simulink model "Mmc"  (R2024b)
settings: Solver=ode23t  StartTime=0.0  StopTime=3  FixedStep=Ts_Power
values from neighbouring files (symbols this model uses):
  alpha_i = (pi/2 - 75/180*pi) / tau_sw    (= 26179.9387799)    [MmcParameters.m]
  C_PM = 6e-3    (= 0.006)    [MmcParameters.m]
  eta = N*delta_wmax*V0^2/(P_rated*sin(phi_r)-Q_rated*cos(phi_r))    [MmcParameters.m]
  Fnom = 50    [MmcParameters.m]
  fs = 400    [MmcParameters.m]
  I_b = Snom/Vnom_AC/sqrt(3)    [MmcParameters.m]
  Ipp_b = Snom/Vnom_AC/sqrt(3/2)    [MmcParameters.m]
  kicir = R0*alpha_ic    (= 2617.99387799)    [MmcParameters.m]
  kiout = R*alpha_i    (= 1308.996939)    [MmcParameters.m]
  kip = 500    [MmcParameters.m]
  kpcir = L0*alpha_ic    (= 416.666666667)    [MmcParameters.m]
  kpout = L*alpha_i    (= 208.333333333)    [MmcParameters.m]
  kpp = 1.5    [MmcParameters.m]
  L = L0/2    (= 0.00795774715459)    [MmcParameters.m]
  L0 = .25 * L_b    (= 0.0159154943092)    [MmcParameters.m]
  mu = eta/2/N/V0^2/(Vmax^2-V0^2)*(P_rated*cos(phi_r)+Q_rated*sin(phi_r))    [MmcParameters.m]
  Nb_PM = 20    [MmcParameters.m]
  phi_r = pi/2    (= 1.57079632679)    [MmcParameters.m]
  R0 = .1    (= 0.1)    [MmcParameters.m]
  SCR = 1.2    [MmcParameters.m]
  SigmaM = 10    [MmcParameters.m]
  Snom = 80e6    (= 80000000)    [MmcParameters.m]
  Ts_Power = 1e-5    (= 1e-05)    [MmcParameters.m]
  V0 = 1    [MmcParameters.m]
  V_b = Vnom_AC    (= 40000)    [MmcParameters.m]
  VDCm = 48e3    (= 48000)    [MmcParameters.m]
  VDCp = 48e3    (= 48000)    [MmcParameters.m]
  Vnom_AC = 40e3    (= 40000)    [MmcParameters.m]
  Vnom_PM = 4.8e3    (= 4800)    [MmcParameters.m]
  w_b = 2*pi*Fnom    (= 314.159265359)    [MmcParameters.m]
undefined symbols (not defined in the file or in its folder): DiscIntNeverNeededParam, Lac, Rac
libraries: spsCurrentMeasurementLib x7, spsHalfBridgeMMCLib x6, spsSeriesRLCBranchLib x6, slpidlib x6, eePwmGeneratorMultilevel x6, spsabctodq0Lib x3, spsMeanLib x2, spsDCVoltageSourceLib x2, spsThreePhaseVIMeasurementLib x2, spsPLL3phLib x2, spsdq0toabcLib x2, spsabctoAlphaBetaZeroLib x2
(part 1 of 2)
settings Model: Creator=The MathWorks, Inc.  LastModifiedBy=smile
settings SolverCC: AlgebraicLoopSolver=TrustRegion
settings DataIOCC: SaveFormat=StructureWithTime  SaveOutput=off  SignalLogging=off  DSMLogging=off  SaveTime=off  ReturnWorkspaceOutputs=off
settings OptimizationCC: ExpressionDepthLimit=2147483647  LifeSpan=inf
settings DebuggingCC: UnderspecifiedInitializationDetection=Classic  MergeDetectMultiDrivingBlocksExec=none  SolverPrmCheckMsg=warning  FcnCallInpInsideContextMsg=warning  UnconnectedInputMsg=warning  UnconnectedOutputMsg=warning  UnconnectedLineMsg=warning  AllowSymbolicDim=off  StateNameClashWarn=warning  SFUnexpectedBacktrackingDiag=warning  SFNoUnconditionalDefaultTransitionDiag=warning  SFExecutionAtInitializationDiag=none  ArithmeticOperatorsInVariantConditions=warning
settings HardwareCC: ProdBitPerPointer=32  ProdBitPerSizeT=32  ProdBitPerPtrDiffT=32  ProdLargestAtomicFloat=None  ProdIntDivRoundTo=Undefined  ProdEndianess=Unspecified  ProdWordSize=32  ProdHWDeviceType=32-bit Generic
settings ModelReferenceCC: EnableRefExpFcnMdlSchedulingChecks=on  PropagateSignalLabelsOutOfModel=off
settings SFSimCC: SimUseLocalCustomCode=off  CustomCodeUndefinedFunction=UseInterfaceOnly
settings RTWCC: RTWUseLocalCustomCode=off  GPUComputeCapability=3.5
settings CodeAppCC: StateflowObjectComments=on
settings GRTTargetCC: TargetLangStandard=C89/C90 (ANSI)  CombineOutputUpdateFcns=off  GRTInterface=on
settings ConfigComp: CovMetricSettings=dw  CovSaveCumulativeToWorkspaceVar=on  CovSaveSingleToWorkspaceVar=on  CovExternalEMLEnable=off
settings SimscapeCC: SimscapeNormalizeSystem=off  SimscapeNominalValues={1, 'bar'; 1, 'cm^3/s'; 1, 'bar*kg/s'; 1, 'kJ/kg'; 1, 'kW'; }

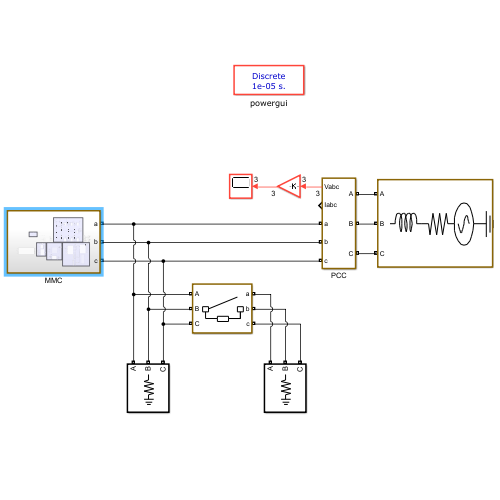
[thumbnail: Simulink's stored preview of the top-level diagram]
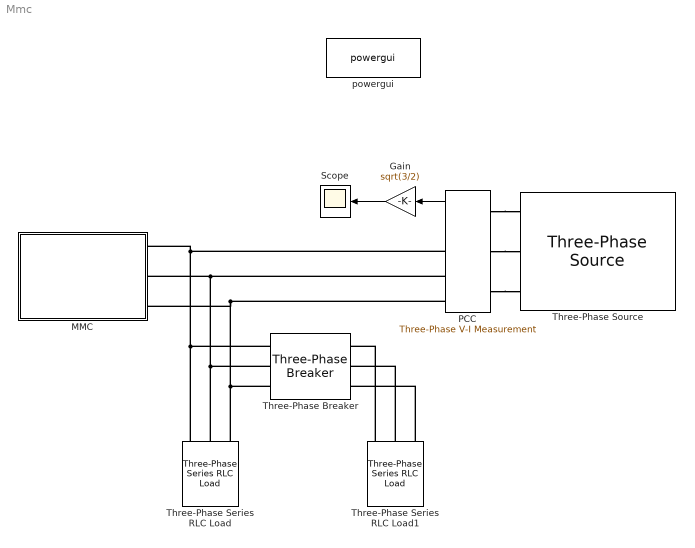
== system Mmc ==
  Gain : Gain  Gain=sqrt(3/2)
  MMC : Subsystem
  PCC : spsThreePhaseVIMeasurementLib/Three-Phase V-I Measurement  VoltageMeasurement=phase-to-ground  SetLabelV=off  LabelV=Vabc  Vpu=off  VpuLL=off  CurrentMeasurement=yes  SetLabelI=off  LabelI=Iabc  Ipu=off  Pbase=Snom  Vbase=Vnom_AC  OutputType=Complex  PhasorSimulation=off  PSBequivalent=0
  Scope : Scope
  Three-Phase Series RLC Load : spsThreePhaseSeriesRLCLoadLib/Three-Phase Series RLC Load  LConnTagsString=A|B|C  Configuration=Y (grounded)  NominalVoltage=Vnom_AC  Vabc=[1e3 1e3 1e3]  Vabcp=[1e3 1e3 1e3]  NominalFrequency=Fnom  UnbalancedPower=off  ActivePower=1e-6  InductivePower=0  CapacitivePower=0  Pabc=[10e3 9e3 11e3]  QLabc=[100 90 110]  QCabc=[100 90 110]  Pabcp=[10e3 9e3 11e3]  QLabcp=[100 90 110]  QCabcp=[100 90 110]  Measurements=None  LoadType=constant Z
  Three-Phase Series RLC Load1 : spsThreePhaseSeriesRLCLoadLib/Three-Phase Series RLC Load  LConnTagsString=A|B|C  Configuration=Y (grounded)  NominalVoltage=Vnom_AC  Vabc=[1e3 1e3 1e3]  Vabcp=[1e3 1e3 1e3]  NominalFrequency=Fnom  UnbalancedPower=off  ActivePower=Snom/1  InductivePower=0  CapacitivePower=0  Pabc=[10e3 9e3 11e3]  QLabc=[100 90 110]  QCabc=[100 90 110]  Pabcp=[10e3 9e3 11e3]  QLabcp=[100 90 110]  QCabcp=[100 90 110]  Measurements=None  LoadType=constant PQ
  Three-Phase Breaker : spsThreePhaseBreakerLib/Three-Phase Breaker  InitialState=open  SwitchA=on  SwitchB=on  SwitchC=on  SwitchTimes=[2]  External=off  BreakerResistance=1e-9  SnubberResistance=1e9  SnubberCapacitance=inf  Measurements=None
  Three-Phase Source : spsThreePhaseSourceLib/Three-Phase Source  InternalConnection=Yg  VoltagePhases=off  Voltage=Vnom_AC/1  PhaseAngle=0  Voltage_phases=[25e3 25e3 25e3]/sqrt(3)  PhaseAngles_phases=[0 -120 +120]  Frequency=Fnom  NonIdealSource=on  SpecifyImpedance=on  Resistance=Rac/1e9  Inductance=Lac/1e4  ShortCircuitLevel=SCR*Snom  BaseVoltage=Vnom_AC  XRratio=7  BusType=swing  Pref=10e3  Qref=0  Prefabc=[10e3, 10e3, 10e3]  Qrefabc=[0, 0, 0]  Qmin=-inf  Qmax=inf
  powergui : sps_lib/powergui  Priority=1  SimulationMode=Discrete  SampleTime=Ts_Power  frequency=60  Iterations=50  frequencyindice=50  Pbase=100e6  ErrMax=1e-4  UnitsV=kV  UnitsW=MW  buscounter=0  FunctionMessages=off  echomessages=off  EnableUseOfTLC=off  CurrentSourceSwitches=off  DisableSnubberDevices=off  DisableRonSwitches=off  DisableVfSwitches=off  DisplayEquations=off  AutomaticDiscreteSolvers=off  SolverType=Tustin/Backward Euler (TBE)  Interpol=off  ExternalGateDelay=off  methode=off  Ts=10  x0status=blocks  SPID=off  SwTol=0  HookPort=off  NonlinearTolerance=1e-4  nMaxIteration=100  ContinueOnMaxIteration=off  RestoreLinks=warning  ResistiveCurrentMeasurement=off  Frange=[0:2:500]  Ylog=off  Xlog=on  ShowGrid=off  save=off  variable=ZData  structure=Vout  ZoomFFT=on  StartTime=0.15  cycles=2  DisplayStyle=1  fundamental=50  FreqAxis=on  MaxFrequency=6000  frequencyindicesteady=1  RmsSteady=1  display=off
  wires:
  PCC/1 -> Gain/1
  Gain/1 -> Scope/1
  connections:
  Three-Phase Series RLC Load/LConn1 -- Three-Phase Breaker/LConn1 -- PCC/RConn1 -- MMC/LConn1
  Three-Phase Series RLC Load/LConn2 -- Three-Phase Breaker/LConn2 -- PCC/RConn2 -- MMC/LConn2
  Three-Phase Series RLC Load/LConn3 -- Three-Phase Breaker/LConn3 -- PCC/RConn3 -- MMC/LConn3
  Three-Phase Series RLC Load1/LConn1 -- Three-Phase Breaker/RConn1
  Three-Phase Series RLC Load1/LConn2 -- Three-Phase Breaker/RConn2
  Three-Phase Series RLC Load1/LConn3 -- Three-Phase Breaker/RConn3
  PCC/LConn1 -- Three-Phase Source/RConn1
  PCC/LConn2 -- Three-Phase Source/RConn2
  PCC/LConn3 -- Three-Phase Source/RConn3

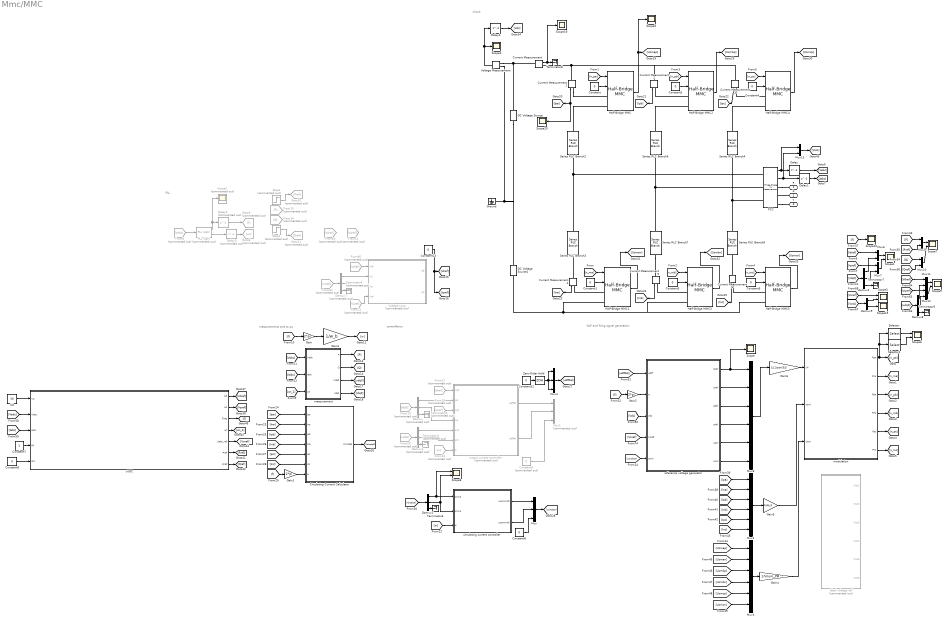
== system Mmc/MMC ==
  note: controllerws
  note: circuit
  note: NLP and firing signal generation
  note: measurements and to pu
  note: PLL
  Circulating Current Calculator : Subsystem
  Constant{,1..6,8,12..13} (10 alike) : Constant  Value=0
  Constant7 : Constant
  Constant9 : Constant  Commented=on  Value=0
  Current Measurement{,1..6} (7 alike) : spsCurrentMeasurementLib/Current Measurement  PhasorSimulation=off  OutputType=Complex  PSBequivalent=0
  DC Voltage Source : spsDCVoltageSourceLib/DC Voltage Source  Amplitude=VDCp  Measurements=None
  DC Voltage Source1 : spsDCVoltageSourceLib/DC Voltage Source  Amplitude=VDCm  Measurements=None
  Delay : Delay  DelayLength=1  SampleTime=Ts_Power
  Delay1 : Delay  DelayLength=1  SampleTime=Ts_Power
  Delay2 : Delay  Commented=on  DelayLength=1  SampleTime=Ts_Power
  Delay3 : Delay  Commented=on  DelayLength=1  SampleTime=Ts_Power
  Delay4 : Delay  DelayLength=1  InputProcessing=Columns as channels (frame based)
  Demux : Demux  Commented=on  Outputs=3
  Demux1 : Demux  Commented=on  Outputs=3
  Demux2 : Demux  Outputs=3
  Demux3 : Demux  Outputs=3
  Demux7 : Demux  Commented=on  Outputs=3
  Demux8 : Demux  Outputs=3
  Demux9 : Demux  Outputs=2
  From13 : From  Commented=on  GotoTag=w
  From15 : From  Commented=on  GotoTag=P
  From16 : From  Commented=on  GotoTag=Q
  From17 : From  Commented=on  GotoTag=idref
  From18 : From  Commented=on  GotoTag=iqref
  From19 : From  Commented=on  GotoTag=idq0
  From20 : From  Commented=on  GotoTag=udq0
  From60 : From  Commented=on  GotoTag=Vdref
  From61 : From  Commented=on  GotoTag=Vqref
  From62 : From  Commented=on  GotoTag=udq0
  From66 : From  Commented=on  GotoTag=Vdref
  From72 : From  Commented=on  GotoTag=Vqref
  From8 : From  Commented=on  GotoTag=Vabc
  Gain : Gain  Gain=2*pi
  Gain1 : Gain  Gain=2*pi
  Gain2 : Gain  Gain=2*pi
  Gain3 : Gain  Gain=1/w_b
  Gain4 : Gain  Gain=1/Vnom_PM
  Gain5 : Gain  Gain=1/Ipp_b
  Gain6 : Gain  Gain=1/1.2/sqrt(3/2)
  Goto10 : Goto  Commented=on  GotoTag=Pref
  Goto11 : Goto  Commented=on  GotoTag=Qref
  Goto8 : Goto  Commented=on  GotoTag=wt
  Goto9 : Goto  Commented=on  GotoTag=f
  Ground : spsGroundLib/Ground  LConnTagsString=a
  Half-Bridge MMC{,1..5} (6 alike) : spsHalfBridgeMMCLib/Half-Bridge MMC  ModelType=Switching devices  n=Nb_PM  C=C_PM  Vc_Initial=Vc_Initial  Ron=Ron  Rs=Rs  Cs=Cs  Ron_Diode=1e-3  Rs_Diode=1e6  Cs_Diode=inf  Vf_Diode=1e-3  Rs_CurrentSource=inf  Ts=10e-6
      settings: LibrarySourceBlock=sps_lib/Power Electronics/Half-Bridge MMC
  Ideal voltage ref : Subsystem  Commented=on
  Mux : Mux  Inputs=3
  Mux1 : Mux  Commented=on  Inputs=3
  Mux{6..7,9..13} (7 alike) : Mux  Inputs=2
  Mux2 : Mux  Inputs=6
  Mux3 : Mux  Inputs=6
  Mux4 : Mux  Inputs=3
  Mux8 : Mux  Inputs=6
  PCC : spsThreePhaseVIMeasurementLib/Three-Phase V-I Measurement  VoltageMeasurement=phase-to-ground  SetLabelV=off  LabelV=Vabc  Vpu=on  VpuLL=off  CurrentMeasurement=yes  SetLabelI=off  LabelI=Iabc  Ipu=on  Pbase=Snom  Vbase=Vnom_AC  OutputType=Complex  PhasorSimulation=off  PSBequivalent=0
  PLL (3ph) : spsPLL3phLib/PLL (3ph)  Commented=on  Fmin=45  Par_Init=[0, 50]  ParK=[9.2/.2 (4.6/.2/.7)^2 0]  TcD=1e-4  MaxRateChangeFreq=12  FilterCutOffFreq=50  Ts=0  AGC=on
  Scope{,4..5,10,15,19..20} (7 alike) : Scope
  Scope{1,3,6..9} (6 alike) : Scope  NumInputPorts=2
  Scope2 : Scope  Commented=on
  Selector : Selector  InputPortWidth=2*Nb_PM  IndexOptions=Index vector (dialog)  Indices=[1]  OutputSizes=1
  Selector1 : Selector  InputPortWidth=2*Nb_PM  IndexOptions=Index vector (dialog)  Indices=[Nb_PM]  OutputSizes=1
  Series RLC Branch{2..4,6..8} (6 alike) : spsSeriesRLCBranchLib/Series RLC Branch  LConnTagsString=__new0  RConnTagsString=__new0  BranchType=RL  Resistance=R0  Inductance=L0  SetiL0=off  InitialCurrent=0  Capacitance=1e-6  Setx0=off  InitialVoltage=0  Measurements=None
  Step2 : Step  Commented=on  Time=.3  Before=-.1  After=.7  SampleTime=Ts_Power
  Step3 : Step  Commented=on  Time=.7  Before=-.1  After=0.7  SampleTime=Ts_Power
  Terminator2 : Terminator  Commented=on
  Terminator3 : Terminator  Commented=on
  Terminator4 : Terminator  Commented=on
  Terminator{6..9} (4 alike) : Terminator
  U0 : Constant  Value=V0  SampleTime=Ts_Power
  Voltage Loop : Subsystem  Commented=on
  Voltage Measurement : spsVoltageMeasurementLib/Voltage Measurement  PhasorSimulation=off  OutputType=Complex  PSBequivalent=0
  Zero-Order Hold : ZeroOrderHold  SampleTime=Ts_Power
  circulating current controller : Subsystem
  measurement : Subsystem
  modulation : Subsystem
  output current controller : Subsystem  Commented=on
  reference voltage generator : Subsystem
  uVOC : Subsystem
  a : PMIOPort  Side=Left
  b : PMIOPort  Port=2  Side=Left
  c : PMIOPort  Port=3  Side=Left
  wires:
  Constant4/1 -> Half-Bridge MMC4/2
  [n_pc] -> Half-Bridge MMC4/1
  [n_pb] -> Half-Bridge MMC2/1
  [n_pa] -> Half-Bridge MMC/1
  [n_mb] -> Half-Bridge MMC3/1
  Constant1/1 -> Half-Bridge MMC1/2
  Constant3/1 -> Half-Bridge MMC3/2
  Half-Bridge MMC/1 -> Scope5/1, [Usmap]
  Constant2/1 -> Half-Bridge MMC2/2
  Constant/1 -> Half-Bridge MMC/2
  [n_ma] -> Half-Bridge MMC1/1
  Constant5/1 -> Half-Bridge MMC5/2
  [n_mc] -> Half-Bridge MMC5/1
  PCC/1 -> Mux13/1, Delay/1
  PCC/2 -> Mux13/2, Delay1/1
  [Vabc] -> measurement/1(Vabc)
  [Iabc] -> measurement/2(Iabc)
  From8/1 -> PLL (3ph)/1
  PLL (3ph)/2 -> Delay3/1
  [wt_2] -> measurement/3(wt)
  PLL (3ph)/1 -> Scope2/1, Delay2/1
  [f] -> Gain/1
  Gain/1 -> Gain3/1
  Gain3/1 -> [w]
  From13/1 -> output current controller/7(w)
  circulating current controller/1(ucommd*) -> Mux/1
  circulating current controller/2(ucommq*) -> Mux/2
  Constant6/1 -> Mux/3
  measurement/1(P) -> [P]
  From17/1 -> output current controller/1(ivd*)
  From18/1 -> output current controller/3(ivq*)
  measurement/3(Vdq0) -> [udq0]
  measurement/4(Idq0) -> [idq0]
  From19/1 -> Demux/1
  Demux/2 -> output current controller/4(ivq)
  Demux/1 -> output current controller/2(ivd)
  Demux/3 -> Terminator2/1
  From20/1 -> Demux1/1
  Demux1/1 -> output current controller/5(uvd)
  Demux1/2 -> output current controller/6(uvq)
  Demux1/3 -> Terminator3/1
  [w] -> circulating current controller/3(w)
  Current Measurement1/1 -> Scope20/1, [Ipa]
  Current Measurement2/1 -> [Ipb]
  Current Measurement3/1 -> [Ipc]
  Current Measurement4/1 -> [Ina]
  Current Measurement5/1 -> [Inb]
  Current Measurement6/1 -> [Inc]
  [Ipa] -> Circulating Current Calculator/1(ipa)
  [Ina] -> Circulating Current Calculator/2(ina)
  [Ipb] -> Circulating Current Calculator/3(ipb)
  [Inb] -> Circulating Current Calculator/4(inb)
  [Ipc] -> Circulating Current Calculator/5(ipc)
  [Inc] -> Circulating Current Calculator/6(inc)
  [f] -> Gain1/1
  Gain1/1 -> Circulating Current Calculator/7(w)
  Circulating Current Calculator/1(icircdq0) -> [Icircdq0]
  [Icircdq0] -> Demux2/1
  Demux2/1 -> Scope8/1, circulating current controller/1(Icircd)
  Demux2/2 -> circulating current controller/2(Icircq), Scope8/2
  Demux2/3 -> Terminator6/1
  Constant9/1 -> Mux1/3
  Gain2/1 -> reference voltage generator/2(w)
  [f] -> Gain2/1
  measurement/2(Q) -> [Q]
  Step3/1 -> Goto11/1
  Delay/1 -> [Vabc]
  Delay1/1 -> [Iabc]
  Delay2/1 -> Goto9/1
  Delay3/1 -> Goto8/1
  modulation/1(Ppa) -> [n_pa], Selector1/1, Selector/1
  modulation/2(Pna) -> [n_ma]
  modulation/3(Ppb) -> [n_pb]
  modulation/4(Pnb) -> [n_mb]
  modulation/5(Ppc) -> [n_pc]
  modulation/6(Pnc) -> [n_mc]
  Step2/1 -> Goto10/1
  [idq0] -> Demux3/1
  Demux3/3 -> Terminator7/1
  [idref] -> Mux6/1
  Demux3/1 -> Mux6/2
  [iqref] -> Mux7/1
  Demux3/2 -> Mux7/2
  Mux/1 -> [ucircdq0]
  [P] -> Mux9/1
  [Pref] -> Mux9/2
  [Q] -> Mux10/1
  [Qref] -> Mux10/2
  reference voltage generator/1(upa*) -> Scope/1, Mux8/1
  reference voltage generator/2(una*) -> Mux8/2
  reference voltage generator/3(upb*) -> Mux8/3
  reference voltage generator/4(unb*) -> Mux8/4
  reference voltage generator/5(upc*) -> Mux8/5
  reference voltage generator/6(unc*) -> Mux8/6
  [Ipa] -> Mux2/1
  [Ina] -> Mux2/2
  [Ipb] -> Mux2/3
  [Inb] -> Mux2/4
  [Ipc] -> Mux2/5
  [Inc] -> Mux2/6
  Mux2/1 -> Gain5/1
  Current Measurement/1 -> Scope19/1, Terminator8/1
  Half-Bridge MMC2/1 -> [Usmbp]
  Half-Bridge MMC4/1 -> [Usmcp]
  Half-Bridge MMC1/1 -> [Usman]
  Half-Bridge MMC3/1 -> [Usmbn]
  Half-Bridge MMC5/1 -> [Usmcn]
  [Usmap] -> Mux3/1
  [Usman] -> Mux3/2
  [Usmbp] -> Mux3/3
  [Usmbn] -> Mux3/4
  [Usmcp] -> Mux3/5
  Mux3/1 -> Gain4/1
  [Usmcn] -> Mux3/6
  Gain4/1 -> modulation/3(Usm)
  Gain5/1 -> modulation/2(Iarm)
  Selector/1 -> Scope6/1
  Selector1/1 -> Scope6/2
  Voltage Measurement/1 -> Delay4/1, Scope4/1
  Delay4/1 -> [Vdc]
  Demux7/1 -> Voltage Loop/2(Vd)
  From62/1 -> Demux7/1
  Demux7/3 -> Terminator4/1
  Demux7/2 -> Voltage Loop/3(Vq)
  From66/1 -> Voltage Loop/1(Vd*)
  Mux6/1 -> Scope1/1
  Mux7/1 -> Scope1/2
  Mux9/1 -> Scope7/1
  Mux10/1 -> Scope7/2
  [udq0] -> Demux8/1
  Demux8/3 -> Terminator9/1
  [Vdref] -> Mux11/1
  Demux8/1 -> Mux11/2
  [Vqref] -> Mux12/1
  Demux8/2 -> Mux12/2
  Mux11/1 -> Scope9/1
  Mux12/1 -> Scope9/2
  Mux13/1 -> [VoIo]
  [VoIo] -> Demux9/1
  [Voref] -> Scope3/1
  Demux9/1 -> Scope3/2
  [f] -> Scope10/1
  From72/1 -> Voltage Loop/4(Vq*)
  [Voref] -> reference voltage generator/4(Voref)
  [ucircdq0] -> reference voltage generator/5(ucirc)
  [udiffdq0] -> reference voltage generator/1(udiff)
  [Vdc] -> reference voltage generator/3(Vdc)
  Demux9/2 -> Scope15/1
  output current controller/1(udiffd*) -> Mux1/1
  output current controller/2(udiffq*) -> Mux1/2
  Mux4/1 -> [udiffdq0]
  Constant13/1 -> [idref], [iqref]
  Mux8/1 -> Gain6/1
  U0/1 -> uVOC/1(V0)
  [Vabc] -> uVOC/2(Vabc)
  [Iabc] -> uVOC/3(Iabc)
  Constant7/1 -> uVOC/4(P0)
  Constant8/1 -> uVOC/5(Q0)
  uVOC/1(Ud) -> [Vdref]
  uVOC/6(Pref) -> [Pref]
  uVOC/2(Uq) -> [Vqref]
  uVOC/3(Freq) -> [f]
  uVOC/4(wt) -> [wt_2]
  uVOC/7(Qref) -> [Qref]
  uVOC/5(Uabc_ref) -> [Voref]
  Gain6/1 -> modulation/1(U*)
  Constant12/1 -> Zero-Order Hold/1
  Zero-Order Hold/1 -> Mux4/3, Mux4/1, Mux4/2
  connections:
  Half-Bridge MMC5/LConn2 -- Half-Bridge MMC3/LConn2 -- Half-Bridge MMC1/LConn2 -- DC Voltage Source1/LConn1
  Series RLC Branch4/LConn1 -- Half-Bridge MMC4/LConn2
  Current Measurement/RConn1 -- Current Measurement2/LConn1 -- Current Measurement3/LConn1 -- Current Measurement1/LConn1
  Series RLC Branch8/LConn1 -- PCC/LConn3 -- Series RLC Branch4/RConn1
  Series RLC Branch2/LConn1 -- Half-Bridge MMC/LConn2
  Series RLC Branch3/LConn1 -- Series RLC Branch2/RConn1 -- PCC/LConn1
  Series RLC Branch6/LConn1 -- Half-Bridge MMC2/LConn2
  Series RLC Branch7/LConn1 -- Series RLC Branch6/RConn1 -- PCC/LConn2
  PCC/RConn1 -- a/RConn1
  b/RConn1 -- PCC/RConn2
  PCC/RConn3 -- c/RConn1
  Current Measurement/LConn1 -- DC Voltage Source/RConn1 -- Voltage Measurement/LConn1
  Current Measurement1/RConn1 -- Half-Bridge MMC/LConn1
  Half-Bridge MMC2/LConn1 -- Current Measurement2/RConn1
  Half-Bridge MMC4/LConn1 -- Current Measurement3/RConn1
  Half-Bridge MMC1/LConn1 -- Current Measurement4/RConn1
  Current Measurement4/LConn1 -- Series RLC Branch3/RConn1
  Series RLC Branch7/RConn1 -- Current Measurement5/LConn1
  Half-Bridge MMC3/LConn1 -- Current Measurement5/RConn1
  Current Measurement6/LConn1 -- Series RLC Branch8/RConn1
  Half-Bridge MMC5/LConn1 -- Current Measurement6/RConn1
  DC Voltage Source1/RConn1 -- DC Voltage Source/LConn1 -- Voltage Measurement/LConn2 -- Ground/LConn1

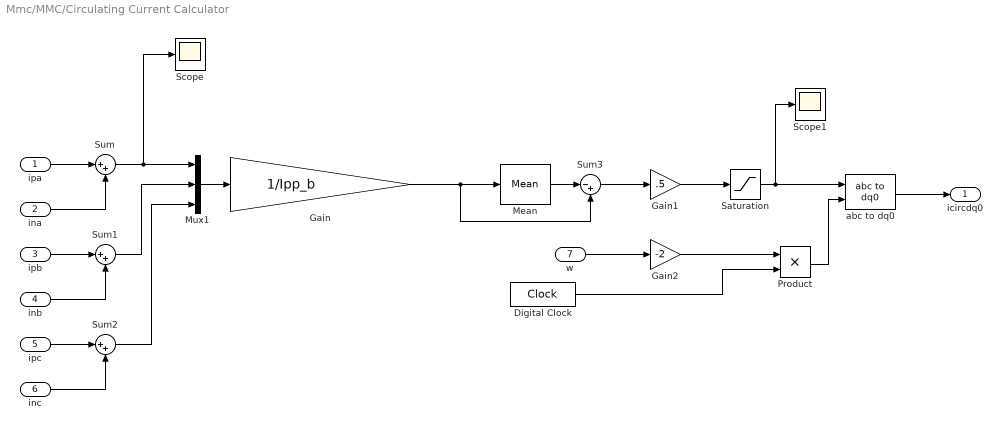
== system Mmc/MMC/Circulating Current Calculator ==
  ipa : Inport
  ina : Inport  Port=2
  ipb : Inport  Port=3
  inb : Inport  Port=4
  ipc : Inport  Port=5
  inc : Inport  Port=6
  w : Inport  Port=7
  Digital Clock : DigitalClock  SampleTime=Ts_Power
  Gain : Gain  Gain=1/Ipp_b
  Gain1 : Gain  Gain=.5
  Gain2 : Gain  Gain=-2
  Mean : spsMeanLib/Mean  Freq=Fnom*2*2  Vinit=0  Ts=Ts_Power
  Mux1 : Mux  Inputs=3
  Product : Product
  Saturation : Saturate  UpperLimit=1.2  LowerLimit=-1.2
  Scope : Scope
  Scope1 : Scope
  Sum : Sum  Inputs=|++
  Sum1 : Sum  Inputs=|++
  Sum2 : Sum  Inputs=|++
  Sum3 : Sum  Inputs=|-+
  abc to dq0 : spsabctodq0Lib/abc to dq0  Alignment=90 degrees behind phase A axis
  icircdq0 : Outport
  wires:
  Sum2/1 -> Mux1/3
  ina/1 -> Sum/2
  Mux1/1 -> Gain/1
  ipb/1 -> Sum1/1
  Sum/1 -> Scope/1, Mux1/1
  Sum1/1 -> Mux1/2
  ipc/1 -> Sum2/1
  inb/1 -> Sum1/2
  ipa/1 -> Sum/1
  inc/1 -> Sum2/2
  Gain1/1 -> Saturation/1
  abc to dq0/1 -> icircdq0/1
  w/1 -> Gain2/1
  Gain2/1 -> Product/1
  Digital Clock/1 -> Product/2
  Product/1 -> abc to dq0/2
  Mean/1 -> Sum3/1
  Sum3/1 -> Gain1/1
  Gain/1 -> Mean/1, Sum3/2
  Saturation/1 -> Scope1/1, abc to dq0/1

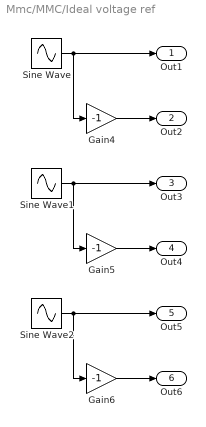
== system Mmc/MMC/Ideal voltage ref ==
  Gain4 : Gain  Gain=-1
  Gain5 : Gain  Gain=-1
  Gain6 : Gain  Gain=-1
  Sine Wave : Sin  Amplitude=sqrt(3/2)  Frequency=50*2*pi  SampleTime=Ts_Power
  Sine Wave1 : Sin  Amplitude=Vnom_AC*sqrt(2/3)/Vnom_PM/Nb_PM  Frequency=50*2*pi  Phase=4*pi/3  SampleTime=Ts_Power
  Sine Wave2 : Sin  Amplitude=Vnom_AC*sqrt(2/3)/Vnom_PM/Nb_PM  Frequency=50*2*pi  Phase=2*pi/3  SampleTime=Ts_Power
  Out1 : Outport
  Out2 : Outport  Port=2
  Out3 : Outport  Port=3
  Out4 : Outport  Port=4
  Out5 : Outport  Port=5
  Out6 : Outport  Port=6
  wires:
  Gain4/1 -> Out2/1
  Sine Wave1/1 -> Out3/1, Gain5/1
  Sine Wave2/1 -> Out5/1, Gain6/1
  Sine Wave/1 -> Out1/1, Gain4/1
  Gain6/1 -> Out6/1
  Gain5/1 -> Out4/1

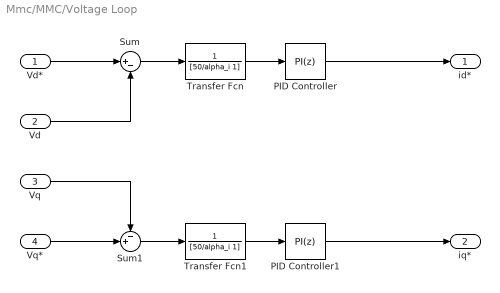
== system Mmc/MMC/Voltage Loop ==
  Vd* : Inport
  Vd : Inport  Port=2
  Vq : Inport  Port=3
  Vq* : Inport  Port=4
  PID Controller : slpidlib/PID Controller  Controller=PI  Form=Parallel  TimeDomain=Discrete-time  UseExternalTs=off  SampleTime=-1  IntegratorMethod=Forward Euler  FilterMethod=Forward Euler  ControllerParametersSource=internal  P=kpp  I=kip  UseKiTs=off  D=0  UseExternalDerivativeSource=off  N=100  UseFilter=on  TunerSelectOption=Transfer Function Based (PID Tuner App)  InitialConditionSource=internal  InitialConditionForIntegrator=0  InitialConditionForFilter=0  DifferentiatorICPrevScaledInput=0  ExternalReset=none  TrackingMode=off  Kt=1  LimitOutput=off  SatLimitsSource=internal  UpperSaturationLimit=inf  LowerSaturationLimit=-inf  LinearizeAsGain=on  AntiWindupMode=none  Kb=1  LimitIntegrator=off  UpperIntegratorSaturationLimit=inf  LowerIntegratorSaturationLimit=-inf  POutMin=[]  POutMax=[]  IOutMin=[]  IOutMax=[]  DOutMin=[]  DOutMax=[]  NOutMin=[]  NOutMax=[]  SumOutMin=[]  SumOutMax=[]  SaturationOutMin=[]  SaturationOutMax=[]  PParamMin=[]  PParamMax=[]  IParamMin=[]  IParamMax=[]  DParamMin=[]  DParamMax=[]  NParamMin=[]  NParamMax=[]  KbParamMin=[]  KbParamMax=[]  KtParamMin=[]  KtParamMax=[]  KbOutMin=[]  KbOutMax=[]  KtOutMin=[]  KtOutMax=[]  IntegratorOutMin=[]  IntegratorOutMax=[]  FilterOutMin=[]  FilterOutMax=[]  SumI1OutMin=[]  SumI1OutMax=[]  SumI2OutMin=[]  SumI2OutMax=[]  SumI3OutMin=[]  SumI3OutMax=[]  SumI4OutMin=[]  SumI4OutMax=[]  SumDOutMin=[]  SumDOutMax=[]  DifferentiatorOutMin=[]  DifferentiatorOutMax=[]  FilterDiffOutCoefMin=[]  FilterDiffOutCoefMax=[]  ReciprocalOutMin=[]  ReciprocalOutMax=[]  SumDenOutMin=[]  SumDenOutMax=[]  SumNumOutMin=[]  SumNumOutMax=[]  DivideOutMin=[]  DivideOutMax=[]  UdiffTsProdOutMin=[]  UdiffTsProdOutMax=[]  NTsProdOutMin=[]  NTsProdOutMax=[]  UintegralTsProdOutMin=[]  UintegralTsProdOutMax=[]  UngainTsProdOutMin=[]  UngainTsProdOutMax=[]  ClampingZeroOutDataTypeStr=Inherit: Inherit via back propagation  ClampingZeroOutMin=[]  ClampingZeroOutMax=[]  FilterDenConstantOutDataTypeStr=Inherit: Inherit via back propagation  FilterDenConstantOutMin=[]  FilterDenConstantOutMax=[]  PCopyOutDataTypeStr=Inherit: Inherit via back propagation  PCopyOutMin=[]  PCopyOutMax=[]  NCopyOutDataTypeStr=Inherit: Inherit via back propagation  NCopyOutMin=[]  NCopyOutMax=[]  IntegratorContinuousStateAttributes=''  IntegratorStateMustResolveToSignalObject=off  IntegratorRTWStateStorageClass=Auto  FilterContinuousStateAttributes=''  FilterStateMustResolveToSignalObject=off  FilterRTWStateStorageClass=Auto  ParallelPVariant=InternalParameters  IdealPVariant=Disabled  IVariant=InternalParameters  DVariant=Disabled  IntegratorVariant=Discrete  SatVariant=Disabled  AWVariant=Passthrough  PCopyVariant=Disabled  TRVariant=Disabled  FdbkBlocksVariant=Forward  IdealPFdbkVariant=Disabled  SatFdbkVariant=Disabled  DerivativeFilterVariant=Disabled  NVariant=Disabled  NCopyVariant=Disabled_SignalSpec  FilterICVariant=Disabled  IntegratorICVariant=InternalICs  ExternalResetVariant=Disabled  TRSumVariant=Passthrough  SumFdbkVariant=Disabled  SumVariant=Sum_PI  TsampFilterVariant=InternalTs  TsampNgainVariant=Passthrough  TsampIntegralVariant=Disabled_SignalSpec  ExternalSaturationOutDataTypeStr=Inherit: Same as second input  DerivativeSourceVariant=Disabled  PreIntVariant=InternalPreInt
  PID Controller1 : slpidlib/PID Controller  Controller=PI  Form=Parallel  TimeDomain=Discrete-time  UseExternalTs=off  SampleTime=-1  IntegratorMethod=Forward Euler  FilterMethod=Forward Euler  ControllerParametersSource=internal  P=kpp  I=kip  UseKiTs=off  D=0  UseExternalDerivativeSource=off  N=100  UseFilter=on  TunerSelectOption=Transfer Function Based (PID Tuner App)  InitialConditionSource=internal  InitialConditionForIntegrator=0  InitialConditionForFilter=0  DifferentiatorICPrevScaledInput=0  ExternalReset=none  TrackingMode=off  Kt=1  LimitOutput=off  SatLimitsSource=internal  UpperSaturationLimit=inf  LowerSaturationLimit=-inf  LinearizeAsGain=on  AntiWindupMode=none  Kb=1  LimitIntegrator=off  UpperIntegratorSaturationLimit=inf  LowerIntegratorSaturationLimit=-inf  POutMin=[]  POutMax=[]  IOutMin=[]  IOutMax=[]  DOutMin=[]  DOutMax=[]  NOutMin=[]  NOutMax=[]  SumOutMin=[]  SumOutMax=[]  SaturationOutMin=[]  SaturationOutMax=[]  PParamMin=[]  PParamMax=[]  IParamMin=[]  IParamMax=[]  DParamMin=[]  DParamMax=[]  NParamMin=[]  NParamMax=[]  KbParamMin=[]  KbParamMax=[]  KtParamMin=[]  KtParamMax=[]  KbOutMin=[]  KbOutMax=[]  KtOutMin=[]  KtOutMax=[]  IntegratorOutMin=[]  IntegratorOutMax=[]  FilterOutMin=[]  FilterOutMax=[]  SumI1OutMin=[]  SumI1OutMax=[]  SumI2OutMin=[]  SumI2OutMax=[]  SumI3OutMin=[]  SumI3OutMax=[]  SumI4OutMin=[]  SumI4OutMax=[]  SumDOutMin=[]  SumDOutMax=[]  DifferentiatorOutMin=[]  DifferentiatorOutMax=[]  FilterDiffOutCoefMin=[]  FilterDiffOutCoefMax=[]  ReciprocalOutMin=[]  ReciprocalOutMax=[]  SumDenOutMin=[]  SumDenOutMax=[]  SumNumOutMin=[]  SumNumOutMax=[]  DivideOutMin=[]  DivideOutMax=[]  UdiffTsProdOutMin=[]  UdiffTsProdOutMax=[]  NTsProdOutMin=[]  NTsProdOutMax=[]  UintegralTsProdOutMin=[]  UintegralTsProdOutMax=[]  UngainTsProdOutMin=[]  UngainTsProdOutMax=[]  ClampingZeroOutDataTypeStr=Inherit: Inherit via back propagation  ClampingZeroOutMin=[]  ClampingZeroOutMax=[]  FilterDenConstantOutDataTypeStr=Inherit: Inherit via back propagation  FilterDenConstantOutMin=[]  FilterDenConstantOutMax=[]  PCopyOutDataTypeStr=Inherit: Inherit via back propagation  PCopyOutMin=[]  PCopyOutMax=[]  NCopyOutDataTypeStr=Inherit: Inherit via back propagation  NCopyOutMin=[]  NCopyOutMax=[]  IntegratorContinuousStateAttributes=''  IntegratorStateMustResolveToSignalObject=off  IntegratorRTWStateStorageClass=Auto  FilterContinuousStateAttributes=''  FilterStateMustResolveToSignalObject=off  FilterRTWStateStorageClass=Auto  ParallelPVariant=InternalParameters  IdealPVariant=Disabled  IVariant=InternalParameters  DVariant=Disabled  IntegratorVariant=Discrete  SatVariant=Disabled  AWVariant=Passthrough  PCopyVariant=Disabled  TRVariant=Disabled  FdbkBlocksVariant=Forward  IdealPFdbkVariant=Disabled  SatFdbkVariant=Disabled  DerivativeFilterVariant=Disabled  NVariant=Disabled  NCopyVariant=Disabled_SignalSpec  FilterICVariant=Disabled  IntegratorICVariant=InternalICs  ExternalResetVariant=Disabled  TRSumVariant=Passthrough  SumFdbkVariant=Disabled  SumVariant=Sum_PI  TsampFilterVariant=InternalTs  TsampNgainVariant=Passthrough  TsampIntegralVariant=Disabled_SignalSpec  ExternalSaturationOutDataTypeStr=Inherit: Same as second input  DerivativeSourceVariant=Disabled  PreIntVariant=InternalPreInt
  Sum : Sum  Inputs=|+-
  Sum1 : Sum  Inputs=-+|
  Transfer Fcn : TransferFcn  Denominator=[50/alpha_i 1]
  Transfer Fcn1 : TransferFcn  Denominator=[50/alpha_i 1]
  id* : Outport
  iq* : Outport  Port=2
  wires:
  Sum/1 -> Transfer Fcn/1
  Sum1/1 -> Transfer Fcn1/1
  Vd*/1 -> Sum/1
  Vd/1 -> Sum/2
  Vq/1 -> Sum1/1
  Vq*/1 -> Sum1/2
  Transfer Fcn/1 -> PID Controller/1
  PID Controller/1 -> id*/1
  Transfer Fcn1/1 -> PID Controller1/1
  PID Controller1/1 -> iq*/1

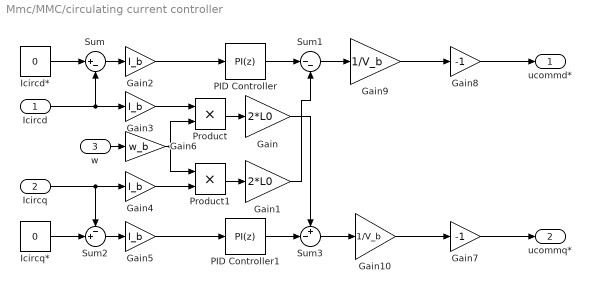
== system Mmc/MMC/circulating current controller ==
  Icircd : Inport
  Icircq : Inport  Port=2
  w : Inport  Port=3
  Gain : Gain  Gain=2*L0
  Gain1 : Gain  Gain=2*L0
  Gain10 : Gain  Gain=1/V_b
  Gain{2..5} (4 alike) : Gain  Gain=I_b
  Gain6 : Gain  Gain=w_b
  Gain7 : Gain  Gain=-1
  Gain8 : Gain  Gain=-1
  Gain9 : Gain  Gain=1/V_b
  Icircd* : Constant  Value=0
  Icircq* : Constant  Value=0
  PID Controller : slpidlib/PID Controller  Controller=PI  Form=Parallel  TimeDomain=Discrete-time  UseExternalTs=off  SampleTime=-1  IntegratorMethod=Forward Euler  FilterMethod=Forward Euler  ControllerParametersSource=internal  P=kpcir  I=kicir  UseKiTs=off  D=0  UseExternalDerivativeSource=off  N=100  UseFilter=on  TunerSelectOption=Transfer Function Based (PID Tuner App)  InitialConditionSource=internal  InitialConditionForIntegrator=0  InitialConditionForFilter=0  DifferentiatorICPrevScaledInput=0  ExternalReset=none  TrackingMode=off  Kt=1  LimitOutput=off  SatLimitsSource=internal  UpperSaturationLimit=inf  LowerSaturationLimit=-inf  LinearizeAsGain=on  AntiWindupMode=none  Kb=1  LimitIntegrator=off  UpperIntegratorSaturationLimit=inf  LowerIntegratorSaturationLimit=-inf  POutMin=[]  POutMax=[]  IOutMin=[]  IOutMax=[]  DOutMin=[]  DOutMax=[]  NOutMin=[]  NOutMax=[]  SumOutMin=[]  SumOutMax=[]  SaturationOutMin=[]  SaturationOutMax=[]  PParamMin=[]  PParamMax=[]  IParamMin=[]  IParamMax=[]  DParamMin=[]  DParamMax=[]  NParamMin=[]  NParamMax=[]  KbParamMin=[]  KbParamMax=[]  KtParamMin=[]  KtParamMax=[]  KbOutMin=[]  KbOutMax=[]  KtOutMin=[]  KtOutMax=[]  IntegratorOutMin=[]  IntegratorOutMax=[]  FilterOutMin=[]  FilterOutMax=[]  SumI1OutMin=[]  SumI1OutMax=[]  SumI2OutMin=[]  SumI2OutMax=[]  SumI3OutMin=[]  SumI3OutMax=[]  SumI4OutMin=[]  SumI4OutMax=[]  SumDOutMin=[]  SumDOutMax=[]  DifferentiatorOutMin=[]  DifferentiatorOutMax=[]  FilterDiffOutCoefMin=[]  FilterDiffOutCoefMax=[]  ReciprocalOutMin=[]  ReciprocalOutMax=[]  SumDenOutMin=[]  SumDenOutMax=[]  SumNumOutMin=[]  SumNumOutMax=[]  DivideOutMin=[]  DivideOutMax=[]  UdiffTsProdOutMin=[]  UdiffTsProdOutMax=[]  NTsProdOutMin=[]  NTsProdOutMax=[]  UintegralTsProdOutMin=[]  UintegralTsProdOutMax=[]  UngainTsProdOutMin=[]  UngainTsProdOutMax=[]  ClampingZeroOutDataTypeStr=Inherit: Inherit via back propagation  ClampingZeroOutMin=[]  ClampingZeroOutMax=[]  FilterDenConstantOutDataTypeStr=Inherit: Inherit via back propagation  FilterDenConstantOutMin=[]  FilterDenConstantOutMax=[]  PCopyOutDataTypeStr=Inherit: Inherit via back propagation  PCopyOutMin=[]  PCopyOutMax=[]  NCopyOutDataTypeStr=Inherit: Inherit via back propagation  NCopyOutMin=[]  NCopyOutMax=[]  IntegratorContinuousStateAttributes=''  IntegratorStateMustResolveToSignalObject=off  IntegratorRTWStateStorageClass=Auto  FilterContinuousStateAttributes=''  FilterStateMustResolveToSignalObject=off  FilterRTWStateStorageClass=Auto  ParallelPVariant=InternalParameters  IdealPVariant=Disabled  IVariant=InternalParameters  DVariant=Disabled  IntegratorVariant=Discrete  SatVariant=Disabled  AWVariant=Passthrough  PCopyVariant=Disabled  TRVariant=Disabled  FdbkBlocksVariant=Forward  IdealPFdbkVariant=Disabled  SatFdbkVariant=Disabled  DerivativeFilterVariant=Disabled  NVariant=Disabled  NCopyVariant=Disabled_SignalSpec  FilterICVariant=Disabled  IntegratorICVariant=InternalICs  ExternalResetVariant=Disabled  TRSumVariant=Passthrough  SumFdbkVariant=Disabled  SumVariant=Sum_PI  TsampFilterVariant=InternalTs  TsampNgainVariant=Passthrough  TsampIntegralVariant=Disabled_SignalSpec  ExternalSaturationOutDataTypeStr=Inherit: Same as second input  DerivativeSourceVariant=Disabled  PreIntVariant=InternalPreInt
  PID Controller1 : slpidlib/PID Controller  Controller=PI  Form=Parallel  TimeDomain=Discrete-time  UseExternalTs=off  SampleTime=-1  IntegratorMethod=Forward Euler  FilterMethod=Forward Euler  ControllerParametersSource=internal  P=kpcir  I=kicir  UseKiTs=off  D=0  UseExternalDerivativeSource=off  N=100  UseFilter=on  TunerSelectOption=Transfer Function Based (PID Tuner App)  InitialConditionSource=internal  InitialConditionForIntegrator=0  InitialConditionForFilter=0  DifferentiatorICPrevScaledInput=0  ExternalReset=none  TrackingMode=off  Kt=1  LimitOutput=off  SatLimitsSource=internal  UpperSaturationLimit=inf  LowerSaturationLimit=-inf  LinearizeAsGain=on  AntiWindupMode=none  Kb=1  LimitIntegrator=off  UpperIntegratorSaturationLimit=inf  LowerIntegratorSaturationLimit=-inf  POutMin=[]  POutMax=[]  IOutMin=[]  IOutMax=[]  DOutMin=[]  DOutMax=[]  NOutMin=[]  NOutMax=[]  SumOutMin=[]  SumOutMax=[]  SaturationOutMin=[]  SaturationOutMax=[]  PParamMin=[]  PParamMax=[]  IParamMin=[]  IParamMax=[]  DParamMin=[]  DParamMax=[]  NParamMin=[]  NParamMax=[]  KbParamMin=[]  KbParamMax=[]  KtParamMin=[]  KtParamMax=[]  KbOutMin=[]  KbOutMax=[]  KtOutMin=[]  KtOutMax=[]  IntegratorOutMin=[]  IntegratorOutMax=[]  FilterOutMin=[]  FilterOutMax=[]  SumI1OutMin=[]  SumI1OutMax=[]  SumI2OutMin=[]  SumI2OutMax=[]  SumI3OutMin=[]  SumI3OutMax=[]  SumI4OutMin=[]  SumI4OutMax=[]  SumDOutMin=[]  SumDOutMax=[]  DifferentiatorOutMin=[]  DifferentiatorOutMax=[]  FilterDiffOutCoefMin=[]  FilterDiffOutCoefMax=[]  ReciprocalOutMin=[]  ReciprocalOutMax=[]  SumDenOutMin=[]  SumDenOutMax=[]  SumNumOutMin=[]  SumNumOutMax=[]  DivideOutMin=[]  DivideOutMax=[]  UdiffTsProdOutMin=[]  UdiffTsProdOutMax=[]  NTsProdOutMin=[]  NTsProdOutMax=[]  UintegralTsProdOutMin=[]  UintegralTsProdOutMax=[]  UngainTsProdOutMin=[]  UngainTsProdOutMax=[]  ClampingZeroOutDataTypeStr=Inherit: Inherit via back propagation  ClampingZeroOutMin=[]  ClampingZeroOutMax=[]  FilterDenConstantOutDataTypeStr=Inherit: Inherit via back propagation  FilterDenConstantOutMin=[]  FilterDenConstantOutMax=[]  PCopyOutDataTypeStr=Inherit: Inherit via back propagation  PCopyOutMin=[]  PCopyOutMax=[]  NCopyOutDataTypeStr=Inherit: Inherit via back propagation  NCopyOutMin=[]  NCopyOutMax=[]  IntegratorContinuousStateAttributes=''  IntegratorStateMustResolveToSignalObject=off  IntegratorRTWStateStorageClass=Auto  FilterContinuousStateAttributes=''  FilterStateMustResolveToSignalObject=off  FilterRTWStateStorageClass=Auto  ParallelPVariant=InternalParameters  IdealPVariant=Disabled  IVariant=InternalParameters  DVariant=Disabled  IntegratorVariant=Discrete  SatVariant=Disabled  AWVariant=Passthrough  PCopyVariant=Disabled  TRVariant=Disabled  FdbkBlocksVariant=Forward  IdealPFdbkVariant=Disabled  SatFdbkVariant=Disabled  DerivativeFilterVariant=Disabled  NVariant=Disabled  NCopyVariant=Disabled_SignalSpec  FilterICVariant=Disabled  IntegratorICVariant=InternalICs  ExternalResetVariant=Disabled  TRSumVariant=Passthrough  SumFdbkVariant=Disabled  SumVariant=Sum_PI  TsampFilterVariant=InternalTs  TsampNgainVariant=Passthrough  TsampIntegralVariant=Disabled_SignalSpec  ExternalSaturationOutDataTypeStr=Inherit: Same as second input  DerivativeSourceVariant=Disabled  PreIntVariant=InternalPreInt
  Product : Product
  Product1 : Product
  Sum : Sum  Inputs=|+-
  Sum1 : Sum  Inputs=|--
  Sum2 : Sum  Inputs=-+|
  Sum3 : Sum  Inputs=+-|
  ucommd* : Outport
  ucommq* : Outport  Port=2
  wires:
  Icircd*/1 -> Sum/1
  Sum/1 -> Gain2/1
  Icircd/1 -> Gain3/1, Sum/2
  Icircq/1 -> Gain4/1, Sum2/1
  Icircq*/1 -> Sum2/2
  Sum2/1 -> Gain5/1
  PID Controller1/1 -> Sum3/2
  PID Controller/1 -> Sum1/1
  w/1 -> Gain6/1
  Product/1 -> Gain/1
  Product1/1 -> Gain1/1
  Sum1/1 -> Gain9/1
  Sum3/1 -> Gain10/1
  Gain/1 -> Sum3/1
  Gain1/1 -> Sum1/2
  Gain2/1 -> PID Controller/1
  Gain3/1 -> Product/1
  Gain6/1 -> Product1/1, Product/2
  Gain4/1 -> Product1/2
  Gain5/1 -> PID Controller1/1
  Gain9/1 -> Gain8/1
  Gain10/1 -> Gain7/1
  Gain8/1 -> ucommd*/1
  Gain7/1 -> ucommq*/1

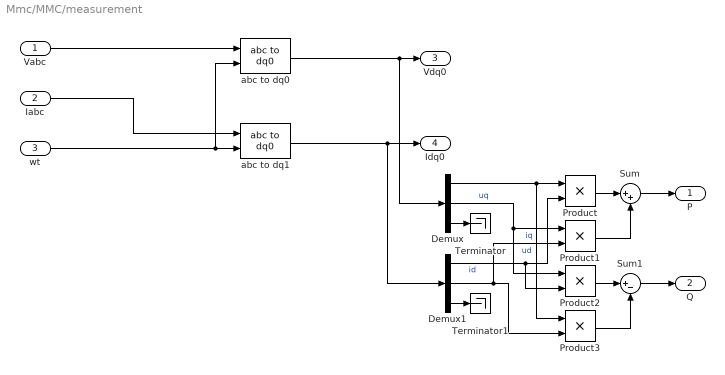
== system Mmc/MMC/measurement ==
  Vabc : Inport
  Iabc : Inport  Port=2
  wt : Inport  Port=3
  Demux : Demux  Outputs=3
  Demux1 : Demux  Outputs=3
  Product{,1..3} (4 alike) : Product
  Sum : Sum  Inputs=|++
  Sum1 : Sum  Inputs=|+-
  Terminator : Terminator
  Terminator1 : Terminator
  abc to dq0 : spsabctodq0Lib/abc to dq0  Alignment=90 degrees behind phase A axis
  abc to dq1 : spsabctodq0Lib/abc to dq0  Alignment=90 degrees behind phase A axis
  P : Outport
  Q : Outport  Port=2
  Vdq0 : Outport  Port=3
  Idq0 : Outport  Port=4
  wires:
  wt/1 -> abc to dq0/2, abc to dq1/2
  Vabc/1 -> abc to dq0/1
  Iabc/1 -> abc to dq1/1
  Demux/3 -> Terminator/1
  Demux1/3 -> Terminator1/1
  Demux/1 -> Product3/1, Product/1  "ud"
  Demux/2 -> Product1/1, Product2/1  "uq"
  Demux1/2 -> Product1/2, Product3/2  "iq"
  Product/1 -> Sum/1
  Product1/1 -> Sum/2
  Product2/1 -> Sum1/1
  Product3/1 -> Sum1/2
  Demux1/1 -> Product2/2, Product/2  "id"
  abc to dq0/1 -> Demux/1, Vdq0/1
  abc to dq1/1 -> Demux1/1, Idq0/1
  Sum/1 -> P/1
  Sum1/1 -> Q/1

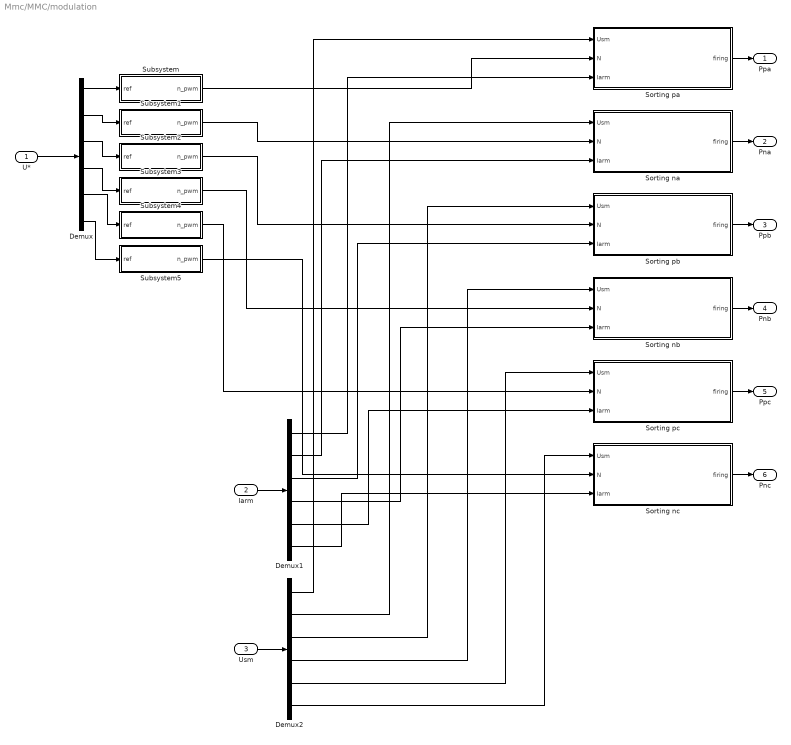
== system Mmc/MMC/modulation ==
  U* : Inport
  Iarm : Inport  Port=2
  Usm : Inport  Port=3
  Demux : Demux  Outputs=6
  Demux1 : Demux  Outputs=6
  Demux2 : Demux  Outputs=6
  Sorting na : Subsystem
  Sorting nb : Subsystem
  Sorting nc : Subsystem
  Sorting pa : Subsystem
  Sorting pb : Subsystem
  Sorting pc : Subsystem
  Subsystem : Subsystem
  Subsystem1 : Subsystem
  Subsystem2 : Subsystem
  Subsystem3 : Subsystem
  Subsystem4 : Subsystem
  Subsystem5 : Subsystem
  Ppa : Outport
  Pna : Outport  Port=2
  Ppb : Outport  Port=3
  Pnb : Outport  Port=4
  Ppc : Outport  Port=5
  Pnc : Outport  Port=6
  wires:
  Demux/2 -> Subsystem1/1(ref)
  Demux/4 -> Subsystem3/1(ref)
  Demux/3 -> Subsystem2/1(ref)
  Demux/6 -> Subsystem5/1(ref)
  Demux/5 -> Subsystem4/1(ref)
  Sorting pa/1(firing) -> Ppa/1
  Sorting na/1(firing) -> Pna/1
  Sorting pb/1(firing) -> Ppb/1
  Sorting nb/1(firing) -> Pnb/1
  Subsystem2/1(n_pwm) -> Sorting pb/2(N)
  Subsystem3/1(n_pwm) -> Sorting nb/2(N)
  Sorting nc/1(firing) -> Pnc/1
  Sorting pc/1(firing) -> Ppc/1
  Subsystem4/1(n_pwm) -> Sorting pc/2(N)
  Subsystem5/1(n_pwm) -> Sorting nc/2(N)
  Iarm/1 -> Demux1/1
  Demux1/1 -> Sorting pa/3(Iarm)
  Demux1/2 -> Sorting na/3(Iarm)
  Demux1/3 -> Sorting pb/3(Iarm)
  Demux1/4 -> Sorting nb/3(Iarm)
  Demux1/5 -> Sorting pc/3(Iarm)
  Demux1/6 -> Sorting nc/3(Iarm)
  Usm/1 -> Demux2/1
  Demux2/6 -> Sorting nc/1(Usm)
  Demux2/5 -> Sorting pc/1(Usm)
  Demux2/4 -> Sorting nb/1(Usm)
  Demux2/3 -> Sorting pb/1(Usm)
  Demux2/2 -> Sorting na/1(Usm)
  Demux2/1 -> Sorting pa/1(Usm)
  U*/1 -> Demux/1
  Subsystem1/1(n_pwm) -> Sorting na/2(N)
  Demux/1 -> Subsystem/1(ref)
  Subsystem/1(n_pwm) -> Sorting pa/2(N)

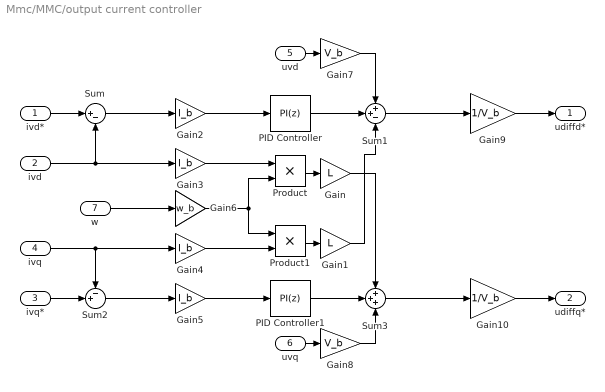
== system Mmc/MMC/output current controller ==
  ivd* : Inport
  ivd : Inport  Port=2
  ivq* : Inport  Port=3
  ivq : Inport  Port=4
  uvd : Inport  Port=5
  uvq : Inport  Port=6
  w : Inport  Port=7
  Gain : Gain  Gain=L
  Gain1 : Gain  Gain=L
  Gain10 : Gain  Gain=1/V_b
  Gain{2..5} (4 alike) : Gain  Gain=I_b
  Gain6 : Gain  Gain=w_b
  Gain7 : Gain  Gain=V_b
  Gain8 : Gain  Gain=V_b
  Gain9 : Gain  Gain=1/V_b
  PID Controller : slpidlib/PID Controller  Controller=PI  Form=Parallel  TimeDomain=Discrete-time  UseExternalTs=off  SampleTime=-1  IntegratorMethod=Forward Euler  FilterMethod=Forward Euler  ControllerParametersSource=internal  P=kpout  I=kiout  UseKiTs=off  D=0  UseExternalDerivativeSource=off  N=100  UseFilter=on  TunerSelectOption=Transfer Function Based (PID Tuner App)  InitialConditionSource=internal  InitialConditionForIntegrator=0  InitialConditionForFilter=0  DifferentiatorICPrevScaledInput=0  ExternalReset=none  TrackingMode=off  Kt=1  LimitOutput=on  SatLimitsSource=internal  UpperSaturationLimit=Vnom_AC*2  LowerSaturationLimit=-Vnom_AC*2  LinearizeAsGain=on  AntiWindupMode=clamping  Kb=1  LimitIntegrator=off  UpperIntegratorSaturationLimit=inf  LowerIntegratorSaturationLimit=-inf  POutMin=[]  POutMax=[]  IOutMin=[]  IOutMax=[]  DOutMin=[]  DOutMax=[]  NOutMin=[]  NOutMax=[]  SumOutMin=[]  SumOutMax=[]  SaturationOutMin=[]  SaturationOutMax=[]  PParamMin=[]  PParamMax=[]  IParamMin=[]  IParamMax=[]  DParamMin=[]  DParamMax=[]  NParamMin=[]  NParamMax=[]  KbParamMin=[]  KbParamMax=[]  KtParamMin=[]  KtParamMax=[]  KbOutMin=[]  KbOutMax=[]  KtOutMin=[]  KtOutMax=[]  IntegratorOutMin=[]  IntegratorOutMax=[]  FilterOutMin=[]  FilterOutMax=[]  SumI1OutMin=[]  SumI1OutMax=[]  SumI2OutMin=[]  SumI2OutMax=[]  SumI3OutMin=[]  SumI3OutMax=[]  SumI4OutMin=[]  SumI4OutMax=[]  SumDOutMin=[]  SumDOutMax=[]  DifferentiatorOutMin=[]  DifferentiatorOutMax=[]  FilterDiffOutCoefMin=[]  FilterDiffOutCoefMax=[]  ReciprocalOutMin=[]  ReciprocalOutMax=[]  SumDenOutMin=[]  SumDenOutMax=[]  SumNumOutMin=[]  SumNumOutMax=[]  DivideOutMin=[]  DivideOutMax=[]  UdiffTsProdOutMin=[]  UdiffTsProdOutMax=[]  NTsProdOutMin=[]  NTsProdOutMax=[]  UintegralTsProdOutMin=[]  UintegralTsProdOutMax=[]  UngainTsProdOutMin=[]  UngainTsProdOutMax=[]  ClampingZeroOutDataTypeStr=Inherit: Inherit via back propagation  ClampingZeroOutMin=[]  ClampingZeroOutMax=[]  FilterDenConstantOutDataTypeStr=Inherit: Inherit via back propagation  FilterDenConstantOutMin=[]  FilterDenConstantOutMax=[]  PCopyOutDataTypeStr=Inherit: Inherit via back propagation  PCopyOutMin=[]  PCopyOutMax=[]  NCopyOutDataTypeStr=Inherit: Inherit via back propagation  NCopyOutMin=[]  NCopyOutMax=[]  IntegratorContinuousStateAttributes=''  IntegratorStateMustResolveToSignalObject=off  IntegratorRTWStateStorageClass=Auto  FilterContinuousStateAttributes=''  FilterStateMustResolveToSignalObject=off  FilterRTWStateStorageClass=Auto  ParallelPVariant=InternalParameters  IdealPVariant=Disabled  IVariant=InternalParameters  DVariant=Disabled  IntegratorVariant=Discrete  SatVariant=Enabled  AWVariant=DiscClampingParallel  PCopyVariant=Disabled  TRVariant=Disabled  FdbkBlocksVariant=Forward  IdealPFdbkVariant=Disabled  SatFdbkVariant=Disabled  DerivativeFilterVariant=Disabled  NVariant=Disabled  NCopyVariant=Disabled_SignalSpec  FilterICVariant=Disabled  IntegratorICVariant=InternalICs  ExternalResetVariant=Disabled  TRSumVariant=Passthrough  SumFdbkVariant=Disabled  SumVariant=Sum_PI  TsampFilterVariant=InternalTs  TsampNgainVariant=Passthrough  TsampIntegralVariant=Disabled_SignalSpec  ExternalSaturationOutDataTypeStr=Inherit: Same as second input  DerivativeSourceVariant=Disabled  PreIntVariant=InternalPreInt
  PID Controller1 : slpidlib/PID Controller  Controller=PI  Form=Parallel  TimeDomain=Discrete-time  UseExternalTs=off  SampleTime=-1  IntegratorMethod=Forward Euler  FilterMethod=Forward Euler  ControllerParametersSource=internal  P=kpout  I=kiout  UseKiTs=off  D=0  UseExternalDerivativeSource=off  N=100  UseFilter=on  TunerSelectOption=Transfer Function Based (PID Tuner App)  InitialConditionSource=internal  InitialConditionForIntegrator=0  InitialConditionForFilter=0  DifferentiatorICPrevScaledInput=0  ExternalReset=none  TrackingMode=off  Kt=1  LimitOutput=on  SatLimitsSource=internal  UpperSaturationLimit=Vnom_AC*2  LowerSaturationLimit=-Vnom_AC*2  LinearizeAsGain=on  AntiWindupMode=clamping  Kb=1  LimitIntegrator=off  UpperIntegratorSaturationLimit=inf  LowerIntegratorSaturationLimit=-inf  POutMin=[]  POutMax=[]  IOutMin=[]  IOutMax=[]  DOutMin=[]  DOutMax=[]  NOutMin=[]  NOutMax=[]  SumOutMin=[]  SumOutMax=[]  SaturationOutMin=[]  SaturationOutMax=[]  PParamMin=[]  PParamMax=[]  IParamMin=[]  IParamMax=[]  DParamMin=[]  DParamMax=[]  NParamMin=[]  NParamMax=[]  KbParamMin=[]  KbParamMax=[]  KtParamMin=[]  KtParamMax=[]  KbOutMin=[]  KbOutMax=[]  KtOutMin=[]  KtOutMax=[]  IntegratorOutMin=[]  IntegratorOutMax=[]  FilterOutMin=[]  FilterOutMax=[]  SumI1OutMin=[]  SumI1OutMax=[]  SumI2OutMin=[]  SumI2OutMax=[]  SumI3OutMin=[]  SumI3OutMax=[]  SumI4OutMin=[]  SumI4OutMax=[]  SumDOutMin=[]  SumDOutMax=[]  DifferentiatorOutMin=[]  DifferentiatorOutMax=[]  FilterDiffOutCoefMin=[]  FilterDiffOutCoefMax=[]  ReciprocalOutMin=[]  ReciprocalOutMax=[]  SumDenOutMin=[]  SumDenOutMax=[]  SumNumOutMin=[]  SumNumOutMax=[]  DivideOutMin=[]  DivideOutMax=[]  UdiffTsProdOutMin=[]  UdiffTsProdOutMax=[]  NTsProdOutMin=[]  NTsProdOutMax=[]  UintegralTsProdOutMin=[]  UintegralTsProdOutMax=[]  UngainTsProdOutMin=[]  UngainTsProdOutMax=[]  ClampingZeroOutDataTypeStr=Inherit: Inherit via back propagation  ClampingZeroOutMin=[]  ClampingZeroOutMax=[]  FilterDenConstantOutDataTypeStr=Inherit: Inherit via back propagation  FilterDenConstantOutMin=[]  FilterDenConstantOutMax=[]  PCopyOutDataTypeStr=Inherit: Inherit via back propagation  PCopyOutMin=[]  PCopyOutMax=[]  NCopyOutDataTypeStr=Inherit: Inherit via back propagation  NCopyOutMin=[]  NCopyOutMax=[]  IntegratorContinuousStateAttributes=''  IntegratorStateMustResolveToSignalObject=off  IntegratorRTWStateStorageClass=Auto  FilterContinuousStateAttributes=''  FilterStateMustResolveToSignalObject=off  FilterRTWStateStorageClass=Auto  ParallelPVariant=InternalParameters  IdealPVariant=Disabled  IVariant=InternalParameters  DVariant=Disabled  IntegratorVariant=Discrete  SatVariant=Enabled  AWVariant=DiscClampingParallel  PCopyVariant=Disabled  TRVariant=Disabled  FdbkBlocksVariant=Forward  IdealPFdbkVariant=Disabled  SatFdbkVariant=Disabled  DerivativeFilterVariant=Disabled  NVariant=Disabled  NCopyVariant=Disabled_SignalSpec  FilterICVariant=Disabled  IntegratorICVariant=InternalICs  ExternalResetVariant=Disabled  TRSumVariant=Passthrough  SumFdbkVariant=Disabled  SumVariant=Sum_PI  TsampFilterVariant=InternalTs  TsampNgainVariant=Passthrough  TsampIntegralVariant=Disabled_SignalSpec  ExternalSaturationOutDataTypeStr=Inherit: Same as second input  DerivativeSourceVariant=Disabled  PreIntVariant=InternalPreInt
  Product : Product
  Product1 : Product
  Sum : Sum  Inputs=|+-
  Sum1 : Sum  Inputs=++-
  Sum2 : Sum  Inputs=-+|
  Sum3 : Sum  Inputs=+++
  udiffd* : Outport
  udiffq* : Outport  Port=2
  wires:
  ivd*/1 -> Sum/1
  ivd/1 -> Gain3/1, Sum/2
  Sum/1 -> Gain2/1
  PID Controller/1 -> Sum1/2
  uvd/1 -> Gain7/1
  Sum1/1 -> Gain9/1
  Sum2/1 -> Gain5/1
  PID Controller1/1 -> Sum3/2
  ivq*/1 -> Sum2/2
  ivq/1 -> Sum2/1, Gain4/1
  uvq/1 -> Gain8/1
  Sum3/1 -> Gain10/1
  Product/1 -> Gain/1
  Product1/1 -> Gain1/1
  Gain3/1 -> Product/1
  Gain4/1 -> Product1/2
  Gain5/1 -> PID Controller1/1
  w/1 -> Gain6/1
  Gain6/1 -> Product/2, Product1/1
  Gain9/1 -> udiffd*/1
  Gain10/1 -> udiffq*/1
  Gain7/1 -> Sum1/1
  Gain8/1 -> Sum3/3
  Gain2/1 -> PID Controller/1
  Gain/1 -> Sum3/1
  Gain1/1 -> Sum1/3

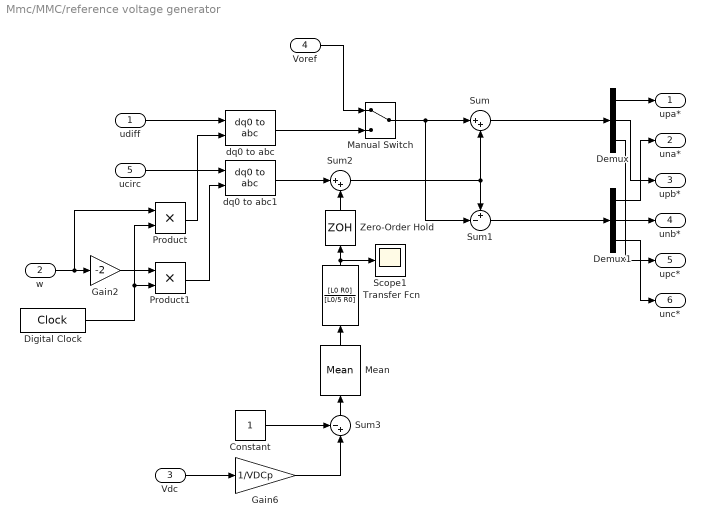
== system Mmc/MMC/reference voltage generator ==
  udiff : Inport
  w : Inport  Port=2
  Vdc : Inport  Port=3
  Voref : Inport  Port=4
  ucirc : Inport  Port=5
  Constant : Constant
  Demux : Demux  Outputs=3
  Demux1 : Demux  Outputs=3
  Digital Clock : DigitalClock  SampleTime=Ts_Power
  Gain2 : Gain  Gain=-2
  Gain6 : Gain  Gain=1/VDCp
  Manual Switch : ManualSwitch
  Mean : spsMeanLib/Mean  Freq=Fnom  Vinit=0  Ts=Ts_Power
  Product : Product
  Product1 : Product
  Scope1 : Scope
  Sum : Sum  Inputs=|++
  Sum1 : Sum  Inputs=+-|
  Sum2 : Sum  Inputs=|++
  Sum3 : Sum  Inputs=-+|
  Transfer Fcn : TransferFcn  Numerator=[L0 R0]  Denominator=[L0/5 R0]
  Zero-Order Hold : ZeroOrderHold  SampleTime=Ts_Power
  dq0 to abc : spsdq0toabcLib/dq0 to abc  Alignment=90 degrees behind phase A axis
  dq0 to abc1 : spsdq0toabcLib/dq0 to abc  Alignment=90 degrees behind phase A axis
  upa* : Outport
  una* : Outport  Port=2
  upb* : Outport  Port=3
  unb* : Outport  Port=4
  upc* : Outport  Port=5
  unc* : Outport  Port=6
  wires:
  Demux/1 -> upa*/1
  Demux/2 -> upb*/1
  Demux/3 -> upc*/1
  Demux1/1 -> una*/1
  Demux1/2 -> unb*/1
  Demux1/3 -> unc*/1
  w/1 -> Product/1, Gain2/1
  Gain2/1 -> Product1/1
  dq0 to abc1/1 -> Sum2/1
  ucirc/1 -> dq0 to abc1/1
  Transfer Fcn/1 -> Zero-Order Hold/1, Scope1/1
  Constant/1 -> Sum3/1
  Sum2/1 -> Sum/2, Sum1/1
  Product1/1 -> dq0 to abc1/2
  Sum3/1 -> Mean/1
  Vdc/1 -> Gain6/1
  Digital Clock/1 -> Product/2, Product1/2
  Product/1 -> dq0 to abc/2
  Gain6/1 -> Sum3/2
  Mean/1 -> Transfer Fcn/1
  Sum1/1 -> Demux1/1
  udiff/1 -> dq0 to abc/1
  Sum/1 -> Demux/1
  Manual Switch/1 -> Sum1/2, Sum/1
  dq0 to abc/1 -> Manual Switch/2
  Voref/1 -> Manual Switch/1
  Zero-Order Hold/1 -> Sum2/2
